simulink model "rete_digitale_in_avanti"  (R2017a)
settings: Solver=FixedStepDiscrete  StartTime=0.0  StopTime=10.0  FixedStep=Tc  RelTol=1e-3
values from neighbouring files (symbols this model uses):
  a1 = 5    [CoeffPerReteDigitale.m]    (also in SistemaDigitaleInAvanti.m = 1000; SistemaDigitaleIndietro.m = 1000)
  a2 = 6    [CoeffPerReteDigitale.m]    (also in SistemaDigitaleInAvanti.m = 1001; SistemaDigitaleIndietro.m = 1001)
  b0 = 0    [CoeffPerReteDigitale.m]    (also in SistemaDigitaleInAvanti.m; SistemaDigitaleIndietro.m)
  b1 = 0    [CoeffPerReteDigitale.m]    (also in SistemaDigitaleInAvanti.m; SistemaDigitaleIndietro.m)
  b2 = 6    [CoeffPerReteDigitale.m]    (also in SistemaDigitaleInAvanti.m = 1000; SistemaDigitaleIndietro.m = 1000)
  Tc = .1    (= 0.1)    [CoeffPerReteDigitale.m]    (also in SistemaDigitaleInAvanti.m = 0.001; SistemaDigitaleIndietro.m = 0.001)
settings Model: Creator=Enrico Donato  LastModifiedBy=Enrico Donato

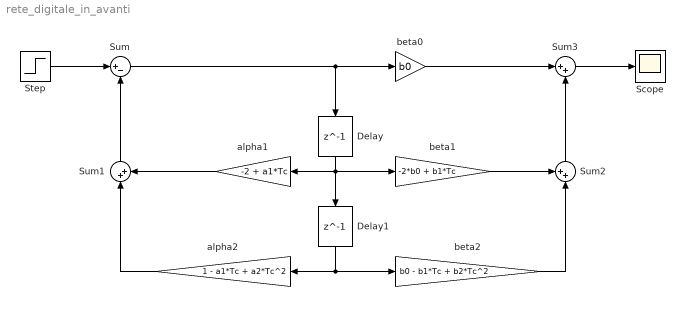
== system rete_digitale_in_avanti ==
  Delay : Delay  DelayLength=1
  Delay1 : Delay  DelayLength=1
  Scope : Scope
  Step : Step  Time=0  SampleTime=Tc
  Sum : Sum  Inputs=|+-
  Sum1 : Sum  Inputs=|++
  Sum2 : Sum  Inputs=++|
  Sum3 : Sum  Inputs=|++
  alpha1 : Gain  Gain=-2 + a1*Tc
  alpha2 : Gain  Gain=1 - a1*Tc + a2*Tc^2
  beta0 : Gain  Gain=b0
  beta1 : Gain  Gain=-2*b0 + b1*Tc
  beta2 : Gain  Gain=b0 - b1*Tc + b2*Tc^2
  wires:
  Delay/1 -> beta1/1, alpha1/1, Delay1/1
  Sum1/1 -> Sum/2
  alpha1/1 -> Sum1/2
  alpha2/1 -> Sum1/1
  Delay1/1 -> alpha2/1, beta2/1
  Sum/1 -> beta0/1, Delay/1
  beta0/1 -> Sum3/1
  beta1/1 -> Sum2/1
  beta2/1 -> Sum2/2
  Sum2/1 -> Sum3/2
  Step/1 -> Sum/1
  Sum3/1 -> Scope/1
